simulink model "Integral_controller_disturbance"  (R2018b)
settings: Solver=VariableStepAuto  StartTime=0.0  StopTime=10  MaxStep=1e-3  RelTol=1e-3
InitFcn:
  | % NOTE: If using VoltPAQ-X1, make sure both Gain switches are set to 3.
  | K_AMP = 3;
  | % Maximum Output Voltage (V): YAW limited to 15 V. PITCH limited to 24 V.
  | VMAX_AMP_P = 24;
  | VMAX_AMP_Y = 15;
  | % Initial Angle of Pitch (rad)
  | theta_0 = -40.5*pi/180;
  | 
  | g = 9.81;
  | 
  | % Pitch and Yaw Motor Armature Resistance (Ohm)
  | R_m_p = 0.83;
  | R_m_y = 1.60;
  | 
  | % Pitch and Yaw Motor Current-Torque Constant (N.m/A)
  | K_t_p = 0.0182;
  | K_t_y = 0.0109;
  | 
  | % Pitch and Yaw Motor Voltage-Torque Constant (N.m/V)
  | K_yp = K_t_p / R_m_p;
  | K_py = K_t_y / R_m_y;
  | 
  | % Pitch and Yaw Viscous Damping Constant (N.m.s/rad)
  | B_p = 0.8;  % tuned while running simulation and experiment in parallel
  | B_y = 0.318; % identified as described in manual
  | 
  | % Mass of the Helicopter (kg)
  | m_heli = 1.3872;
  | 
  | % Mass of the Helicopter with Yoke (kg)
  | m_heli_case = 1.421;
  | 
  | % Distance from Pitch Pivot to Pitch/Front Motor and Yaw/Back Motor(m)
  | r_p = 7.75*0.0254;
  | r_y = (6+5/8)*0.0254;
  | 
  | % Pitch and Yaw Propeller Force-Thrust Constant found Experimentally (N/V)
  | K_f_p = 5*0.2074;
  | K_f_y = 3*0.1426;
  | 
  | % Pitch and Yaw Propeller Torque-Thrust Constant found Experimentally (N.m/V)
  | K_pp = K_f_p * r_p;
  | K_yy = K_f_y * r_y;
  | 
  | % Mass of Pitch/Front Motor and Yaw/Back Motor (kg)
  | m_motor_p = 0.292;
  | m_motor_y = 0.128;
  | 
  | % Mass of Pitch/Front and Yaw/Back Guard + Propeller(kg)
  | m_shield = 0.143 + 0.024;
  | 
  | % Total Mass of Pitch and Yaw Motor/Shield Assemblies (kg)
  | m_props = ( m_motor_p + m_motor_y + 2 * m_shield );
  | 
  | % Mass of Helicopter Body moving about Pitch Axis (kg)
  | m_body_p = m_heli - m_props;
  | 
  | % Mass of Helicopter Body moving about Yaw Axis (kg)
  | m_body_y = m_heli_case - m_props;
  | 
  | % Mass of Metal Shaft Moving about Yaw Axis (kg)
  | m_shaft = 0.151;
  | 
  | % Total Length of Helicopter Body (m)
  | L_body = 19*0.0254;
  | 
  | % Helicopter Center of Mass from Pivot along Pitch Axis (m)
  | l_cm = ( (m_motor_p + m_shield ) * r_p +  (m_motor_y + m_shield ) * r_y ) / ( m_props ) ;
  | 
  | % Length of Metal Shaft Moving about Yaw Axis through slip ring (m)
  | L_shaft = 11 * 0.0254;
  | 
  | % Pitch and Yaw Motor Rotor Moment of Inertia (kg.m^2)
  | J_m_p = 1.91e-6; %1.7070e-5;
  | J_m_y = 1.374e-4; %1.4471e-5;
  | 
  | % Moment of Inertia of Helicopter Body about its CM (kg.m^2)
  | J_body_p = m_body_p * L_body^2 / 12;
  | J_body_y = m_body_y * L_body^2 / 12;
  | 
  | % Moment of Inertia of Metal Shaft about Yaw Axis (kg.m^2)
  | J_shaft = m_shaft * L_shaft^2 / 3; %;0.0851;
  | 
  | % Moment of Inertia of Pitch Motor + Guard Assembly about Pivot (kg.m^2)
  | J_p = ( m_motor_p + m_shield ) * r_p^2;
  | 
  | % Moment of Inertia of Yaw Motor + Guard Assembly about Pivot (kg.m^2)
  | J_y = ( m_motor_y + m_shield ) * r_y^2;
  | 
  | % Equivalent Moment of Inertia about Pitch and Yaw Axis (kg.m^2)
  | J_eq_p = J_m_p + J_body_p + J_p + J_y;
  | J_eq_y = J_m_y + J_body_y + J_p + J_y + J_shaft;
  | 
  | 
  | %BESSEL wn=4
  | Kbes=[     68.5119  -25.1203    5.3421   -3.6881
  |    63.1652  188.4894    0.7783   19.4789];
  | 
  | xd=-20;
libraries: simulink x1
settings Model: Creator=rezan  LastModifiedBy=rezan
settings DataIOCC: ReturnWorkspaceOutputs=on
settings DebuggingCC: UnconnectedInputMsg=none  UnconnectedOutputMsg=none  UnconnectedLineMsg=none  SFMachineParentedDataDiag=error

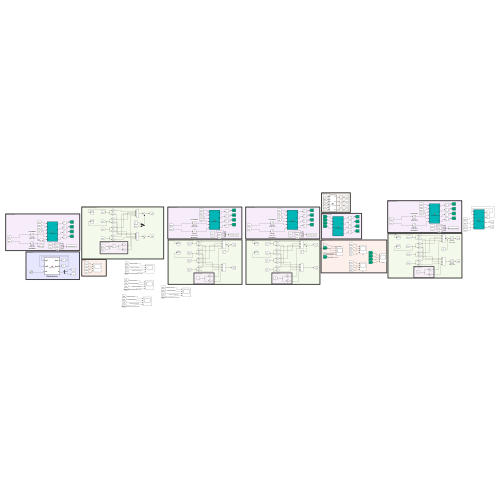
[thumbnail: Simulink's stored preview of the top-level diagram]
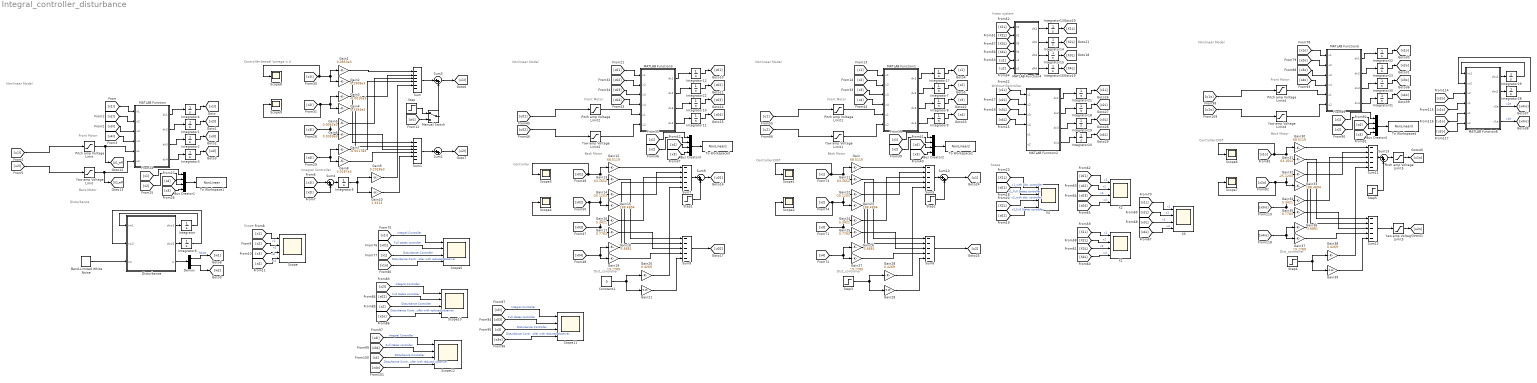
== system Integral_controller_disturbance ==
  note: Scope
  note: Disturbance
  note: Integral Controller
  note: Controller-bessel \omega = 4
  note: Front Motor
  note: Back Motor
  note: Nonlinear Model
  note: Controller-DIST
  note: Back Motor
  note: Dist_controller
  note: Scope
  note: Nonlinear Model
  note: Front Motor
  note: linear system
  note: Without Controller
  note: Dist_controller
  note: Controller
  note: Back Motor
  note: Nonlinear Model
  note: Front Motor
  note: Controller-DIST
  note: Dist_controller
  note: Front Motor
  note: Back Motor
  note: Nonlinear Model
  Band-Limited White Noise : simulink/Sources/Band-Limited White Noise  Cov=5  Ts=0.1  seed=[23341]
  Bus Creator{1..4} (4 alike) : BusCreator  Inputs=4
  Constant1 : Constant  Value=0
  Demux : Demux  Outputs=2
  Disturbance : MATLAB Function  TreatAsAtomicUnit=on
  Gain : Gain  Gain=68.5119
  Gain1 : Gain  Gain=0.0853e3
  Gain10 : Gain  Gain=1.3313
  Gain11 : Gain  Gain=63.1652
  Gain12 : Gain  Gain=68.5119
  Gain13 : Gain  Gain=63.1652
  Gain14 : Gain  Gain=-25.1203
  Gain15 : Gain  Gain=188.4894
  Gain16 : Gain  Gain=5.3421
  Gain17 : Gain  Gain=0.7783
  Gain18 : Gain  Gain=-3.6881
  Gain19 : Gain  Gain=19.4789
  Gain2 : Gain  Gain=0.1908e3
  Gain20 : Gain  Gain=0.4269
  Gain21 : Gain  Gain=-0.13
  Gain22 : Gain  Gain=-25.1203
  Gain23 : Gain  Gain=188.4894
  Gain24 : Gain  Gain=5.3421
  Gain25 : Gain  Gain=0.7783
  Gain26 : Gain  Gain=-3.6881
  Gain27 : Gain  Gain=19.4789
  Gain28 : Gain  Gain=0.4269
  Gain29 : Gain  Gain=-0.13
  Gain3 : Gain  Gain=-0.0010e3
  Gain30 : Gain  Gain=68.5119
  Gain31 : Gain  Gain=63.1652
  Gain32 : Gain  Gain=-25.1203
  Gain33 : Gain  Gain=188.4894
  Gain34 : Gain  Gain=5.3421
  Gain35 : Gain  Gain=0.7783
  Gain36 : Gain  Gain=-3.6881
  Gain37 : Gain  Gain=19.4789
  Gain38 : Gain  Gain=0.4269
  Gain39 : Gain  Gain=-0.13
  Gain4 : Gain  Gain=0.3394e3
  Gain5 : Gain  Gain=0.0061e3
  Gain6 : Gain  Gain=0.0059e3
  Gain7 : Gain  Gain=-0.0017e3
  Gain8 : Gain  Gain=0.0287e3
  Gain9 : Gain  Gain=0.2028e3
  Integrator{,1,3,6..7,9,11,14,16,18,20,22..23,28..29,31} (16 alike) : Integrator
  Integrator{2,8,10,15,19,30} (6 alike) : Integrator  InitialCondition=10
  Integrator{4..5,12..13,17,21,32} (7 alike) : Integrator  UpperSaturationLimit=40.5*pi/180  LowerSaturationLimit=-40.5*pi/180
  MATLAB Function : MATLAB Function  TreatAsAtomicUnit=on
  MATLAB Function1 : MATLAB Function  TreatAsAtomicUnit=on
  MATLAB Function2 : MATLAB Function  TreatAsAtomicUnit=on
  MATLAB Function3 : MATLAB Function  TreatAsAtomicUnit=on
  MATLAB Function4 : MATLAB Function  TreatAsAtomicUnit=on
  MATLAB Function5 : MATLAB Function  TreatAsAtomicUnit=on
  MATLAB Function8 : MATLAB Function  TreatAsAtomicUnit=on
  Manual Switch : ManualSwitch
  Pitch amp Voltage Limit{,1..2,4..5} (5 alike) : Saturate  UpperLimit=VMAX_AMP_P  LowerLimit=- VMAX_AMP_P
  Scope{,5,10..12} (5 alike) : Scope  NumInputPorts=4
  Scope{1..4,6..9} (8 alike) : Scope
  Step{,1..5} (6 alike) : Step  SampleTime=0
  Sum : Sum  Inputs=------
  Sum1 : Sum  Inputs=------
  Sum{2..4,9..10,13} (6 alike) : Sum  Inputs=|++
  Sum{5..8,11..12} (6 alike) : Sum  Inputs=-----
  To Workspace1 : ToWorkspace  VariableName=NonLinear  SampleTime=-1
  To Workspace2 : ToWorkspace  VariableName=NonLinear2  SampleTime=-1
  To Workspace3 : ToWorkspace  VariableName=NonLinear1  SampleTime=-1
  To Workspace4 : ToWorkspace  VariableName=NonLinear3  SampleTime=-1
  X{1..4} (4 alike) : Scope  NumInputPorts=4
  Yaw amp Voltage Limit{,1..2,4..5} (5 alike) : Saturate  UpperLimit=VMAX_AMP_Y  LowerLimit=- VMAX_AMP_Y
  wires:
  Sum1/1 -> Sum2/1
  Gain4/1 -> Sum1/2
  [x2I] -> Scope9/1, Gain3/1, Gain4/1
  Integrator5/1 -> Gain10/1, Gain9/1
  Gain6/1 -> Sum1/3
  Sum3/1 -> [u1I]
  Gain7/1 -> Sum/4
  [x4I] -> Gain8/1, Gain7/1
  Gain2/1 -> Sum1/1
  Gain9/1 -> Sum/5
  Gain5/1 -> Sum/3
  [x3I] -> Gain5/1, Gain6/1
  Sum2/1 -> [u2I]
  Sum/1 -> Sum3/1
  Gain1/1 -> Sum/1
  Gain8/1 -> Sum1/4
  [x1I] -> Scope8/1, Gain2/1, Gain1/1
  Gain10/1 -> Sum1/5
  Gain3/1 -> Sum/2
  MATLAB Function/3(dx3) -> Integrator2/1
  Integrator4/1 -> [x1I]
  [x2] -> Bus Creator1/2
  Pitch amp Voltage Limit/1 -> [U1_eff], MATLAB Function/5(u1)
  Bus Creator1/1 -> To Workspace1/1
  [x4] -> Bus Creator1/3
  [x3I] -> MATLAB Function/3(x3)
  Integrator2/1 -> [x3I]
  MATLAB Function/1(dx1) -> Integrator4/1
  MATLAB Function/4(dx4) -> Integrator3/1
  MATLAB Function/2(dx2) -> Integrator1/1
  [x2I] -> MATLAB Function/2(x2)
  [u1I] -> Pitch amp Voltage Limit/1
  Integrator3/1 -> [x4I]
  [u2I] -> Yaw amp Voltage Limit/1
  [x4I] -> MATLAB Function/4(x4)
  [x3] -> Bus Creator1/4
  [x1] -> Bus Creator1/1
  Integrator1/1 -> [x2I]
  Yaw amp Voltage Limit/1 -> [U2_eff], MATLAB Function/6(u2)
  [x1I] -> MATLAB Function/1(x1)
  [x1I] -> Sum4/1
  [x2I] -> Sum4/2
  Sum4/1 -> Integrator5/1
  [x1] -> Scope/1  "x1"
  [x2] -> Scope/2  "x2"
  [x3] -> Scope/3  "x3"
  [x4] -> Scope/4  "x4"
  Disturbance/1(dxw1) -> Integrator/1
  Band-Limited White Noise/1 -> Disturbance/3(uw)
  Integrator/1 -> Disturbance/1(xw1)
  Disturbance/2(dxw2) -> Integrator6/1
  Integrator6/1 -> Disturbance/2(xw2)
  Demux/1 -> [w1]  "Noise"
  Disturbance/3(w) -> Demux/1
  Demux/2 -> [w2]
  Step/1 -> Manual Switch/1
  [w1] -> Manual Switch/2
  Manual Switch/1 -> Sum3/2
  [X2L] -> MATLAB Function4/2(X2)
  [x1] -> Bus Creator3/1
  Integrator15/1 -> [X3L]
  Sum10/1 -> [u1]
  Integrator14/1 -> [X2L]
  [u1] -> MATLAB Function4/5(u1)
  [x4] -> MATLAB Function1/4(x4)
  [x04] -> MATLAB Function3/4(x4)
  [X1L] -> MATLAB Function4/1(X1)
  [X2L] -> X1/2  "x2"
  [x3] -> Bus Creator3/4
  Gain17/1 -> Sum8/3
  Yaw amp Voltage Limit1/1 -> MATLAB Function1/6(u2)
  Integrator16/1 -> [X4L]
  Integrator13/1 -> [X1L]
  Integrator10/1 -> [x03]
  Integrator12/1 -> [x01]
  [x02] -> X4/4  "x2_Full States controller"
  MATLAB Function2/1(dx1) -> Integrator21/1
  Integrator21/1 -> [x1L]
  Gain22/1 -> Sum5/2
  [x01] -> Gain12/1, Gain13/1, Scope3/1
  [x2] -> Scope2/1, Gain22/1, Gain23/1
  Constant1/1 -> Gain20/1, Gain21/1
  MATLAB Function4/2(dX2) -> Integrator14/1
  Bus Creator3/1 -> To Workspace3/1
  [X4L] -> MATLAB Function4/4(X4)
  Gain12/1 -> Sum7/1
  [x1L] -> MATLAB Function2/1(x1)
  [X3L] -> MATLAB Function4/3(X3)
  MATLAB Function4/1(dX1) -> Integrator13/1
  Integrator22/1 -> [x02]
  [u01] -> Pitch amp Voltage Limit2/1
  [x4] -> Bus Creator3/3
  [x01] -> MATLAB Function3/1(x1)
  Yaw amp Voltage Limit2/1 -> MATLAB Function3/6(u2)
  [u02] -> Yaw amp Voltage Limit2/1
  [x2] -> MATLAB Function1/2(x2)
  Integrator11/1 -> [x04]
  MATLAB Function3/3(dx3) -> Integrator10/1
  [x3] -> MATLAB Function1/3(x3)
  Integrator20/1 -> [x4L]
  MATLAB Function1/4(dx4) -> Integrator9/1
  [x04] -> Gain18/1, Gain19/1
  MATLAB Function3/2(dx2) -> Integrator22/1
  [x03] -> MATLAB Function3/3(x3)
  Gain13/1 -> Sum8/1
  Gain18/1 -> Sum7/4
  Gain15/1 -> Sum8/2
  MATLAB Function3/1(dx1) -> Integrator12/1
  Gain16/1 -> Sum7/3
  [x02] -> Gain15/1, Gain14/1, Scope4/1
  Gain27/1 -> Sum6/4
  Sum8/1 -> [u02]
  MATLAB Function2/4(dx4) -> Integrator20/1
  MATLAB Function1/3(dx3) -> Integrator8/1
  Bus Creator2/1 -> To Workspace2/1
  MATLAB Function2/3(dx3) -> Integrator19/1
  Integrator19/1 -> [x3L]
  [x3L] -> MATLAB Function2/3(x3)
  Gain11/1 -> Sum6/1
  [x4L] -> MATLAB Function2/4(x4)
  [x4] -> Gain27/1, Gain26/1
  Gain28/1 -> Sum5/5
  Gain25/1 -> Sum6/3
  MATLAB Function4/4(dX4) -> Integrator16/1
  [u1] -> Pitch amp Voltage Limit1/1
  Integrator18/1 -> [x2L]
  [x1] -> Scope1/1, Gain11/1, Gain/1
  Integrator9/1 -> [x4]
  [x2] -> Bus Creator3/2
  Gain/1 -> Sum5/1
  [x2] -> Bus Creator2/2
  MATLAB Function2/2(dx2) -> Integrator18/1
  [X2L] -> X4/3  "x2_with dist. controller"
  [x1] -> Bus Creator2/1
  [x3] -> Gain24/1, Gain25/1
  MATLAB Function1/1(dx1) -> Integrator17/1
  [x1] -> MATLAB Function1/1(x1)
  [X3L] -> X1/3  "x3"
  [X1L] -> X4/1  "x1_with dist. controller"
  [u2] -> Yaw amp Voltage Limit1/1
  Integrator8/1 -> [x3]
  [x02] -> X2/2  "x2"
  [x03] -> X2/3  "x3"
  Pitch amp Voltage Limit1/1 -> MATLAB Function1/5(u1)
  Gain19/1 -> Sum8/4
  [x01] -> X2/1  "x1"
  [X1L] -> X1/1  "x1"
  MATLAB Function4/3(dX3) -> Integrator15/1
  Gain29/1 -> Sum6/5
  Integrator7/1 -> [x2]
  [x01] -> X4/2  "x1_Full States controller"
  MATLAB Function3/4(dx4) -> Integrator11/1
  Gain26/1 -> Sum5/4
  [x02] -> MATLAB Function3/2(x2)
  Gain14/1 -> Sum7/2
  Gain23/1 -> Sum6/2
  [x4L] -> X3/4  "x4"
  [X4L] -> X1/4  "x4"
  Step3/1 -> Gain29/1, Gain28/1
  Gain20/1 -> Sum7/5
  Integrator17/1 -> [x1]
  Sum6/1 -> [u2]
  Gain24/1 -> Sum5/3
  [x1L] -> X3/1  "x1"
  MATLAB Function1/2(dx2) -> Integrator7/1
  [x03] -> Gain17/1, Gain16/1
  [x04] -> X2/4  "x4"
  Gain21/1 -> Sum8/5
  [x4] -> Bus Creator2/3
  [x2L] -> X3/2  "x2"
  [x3L] -> X3/3  "x3"
  [x3] -> Bus Creator2/4
  Pitch amp Voltage Limit2/1 -> MATLAB Function3/5(u1)
  [x2L] -> MATLAB Function2/2(x2)
  [u2] -> MATLAB Function4/6(u2)
  Step1/1 -> Sum9/2
  Sum9/1 -> [u01]
  Sum7/1 -> Sum9/1
  Sum5/1 -> Sum10/1
  Step2/1 -> Sum10/2
  [x1I] -> Scope5/1  "Integral Controller"
  [x01] -> Scope5/2  "Full states controller"
  [x1] -> Scope5/3  "Disturbance Controller"
  Step4/1 -> Gain39/1, Gain38/1
  Gain38/1 -> Sum11/5
  [x4o] -> MATLAB Function5/4(x4)
  [x2o] -> Scope7/1, Gain32/1, Gain33/1
  Integrator30/1 -> [x3o]
  [x3o] -> MATLAB Function5/3(x3)
  [x1o] -> Scope6/1, Gain31/1, Gain30/1
  [u1o] -> Pitch amp Voltage Limit4/1
  MATLAB Function5/2(dx2) -> Integrator23/1
  Integrator31/1 -> [x4o]
  Integrator32/1 -> [x1o]
  Sum12/1 -> Yaw amp Voltage Limit5/1
  Gain35/1 -> Sum12/3
  Gain33/1 -> Sum12/2
  Gain34/1 -> Sum11/3
  Gain30/1 -> Sum11/1
  [x3ro] -> Gain34/1, Gain35/1
  Gain39/1 -> Sum12/5
  [x2o] -> MATLAB Function8/3(x2)
  [u2o] -> MATLAB Function8/6(u2)
  Gain36/1 -> Sum11/4
  Integrator28/1 -> MATLAB Function8/2(xc2)
  [x2] -> Bus Creator4/2
  MATLAB Function8/1(dxc1) -> Integrator29/1
  Integrator29/1 -> MATLAB Function8/1(xc1)
  [x4ro] -> Gain37/1, Gain36/1
  MATLAB Function8/2(dxc2) -> Integrator28/1
  MATLAB Function5/4(dx4) -> Integrator31/1
  MATLAB Function5/1(dx1) -> Integrator32/1
  Yaw amp Voltage Limit4/1 -> MATLAB Function5/6(u2)
  [x3] -> Bus Creator4/4
  MATLAB Function5/3(dx3) -> Integrator30/1
  Gain32/1 -> Sum11/2
  Pitch amp Voltage Limit5/1 -> [u1o]
  MATLAB Function8/4(x1e) -> [x3ro]  "x1e"
  Yaw amp Voltage Limit5/1 -> [u2o]
  [x1] -> Bus Creator4/1
  [u1o] -> MATLAB Function8/5(u1)
  Integrator23/1 -> [x2o]
  [x1o] -> MATLAB Function8/4(x1)
  [x2o] -> MATLAB Function5/2(x2)
  [u2o] -> Yaw amp Voltage Limit4/1
  [x1o] -> MATLAB Function5/1(x1)
  Gain37/1 -> Sum12/4
  MATLAB Function8/3(x2e) -> [x4ro]  "x2e"
  [x4] -> Bus Creator4/3
  Bus Creator4/1 -> To Workspace4/1
  Pitch amp Voltage Limit4/1 -> MATLAB Function5/5(u1)
  Gain31/1 -> Sum12/1
  Step5/1 -> Sum13/2
  Sum11/1 -> Sum13/1
  Sum13/1 -> Pitch amp Voltage Limit5/1
  [x1o] -> Scope5/4  "Disturbance Controller with reduced observer"
  [x2o] -> Scope10/4  "Disturbance Controller with reduced observer"
  [x2] -> Scope10/3  "Disturbance Controller"
  [x02] -> Scope10/2  "Full states controller"
  [x2I] -> Scope10/1  "Integral Controller"
  [x3I] -> Scope11/1  "Integral Controller"
  [x03] -> Scope11/2  "Full states controller"
  [x3] -> Scope11/3  "Disturbance Controller"
  [x3o] -> Scope11/4  "Disturbance Controller with reduced observer"
  [x4o] -> Scope12/4  "Disturbance Controller with reduced observer"
  [x4] -> Scope12/3  "Disturbance Controller"
  [x04] -> Scope12/2  "Full states controller"
  [x4I] -> Scope12/1  "Integral Controller"

== matlab function Integral_controller_disturbance/MATLAB Function1 ==
  data: x1 input; x2 input; x3 input; x4 input; u1 input; dx1 output; u2 input; dx2 output; dx3 output; dx4 output
function [dx1,dx2,dx3,dx4]= NonlinearFunc(x1,x2,x3,x4,u1,u2)
%% Initial Conditions
% Gravitational Constant (m/s^2)
g = 9.81;

% Pitch and Yaw Motor Armature Resistance (Ohm)
R_m_p = 0.83;
R_m_y = 1.60;

% Pitch and Yaw Motor Current-Torque Constant (N.m/A)
K_t_p = 0.0182;
K_t_y = 0.0109;

% Pitch and Yaw Motor Voltage-Torque Constant (N.m/V)
K_yp = K_t_p / R_m_p;
K_py = K_t_y / R_m_y;

% Pitch and Yaw Viscous Damping Constant (N.m.s/rad)
B_p = 0.8;  % tuned while running simulation and experiment in parallel
B_y = 0.318; % identified as described in manual 

% Mass of the Helicopter (kg)
m_heli = 1.3872;

% Mass of the Helicopter with Yoke (kg)
m_heli_case = 1.421;

% Distance from Pitch Pivot to Pitch/Front Motor and Yaw/Back Motor(m)
r_p = 7.75*0.0254;
r_y = (6+5/8)*0.0254;

% Pitch and Yaw Propeller Force-Thrust Constant found Experimentally (N/V)
K_f_p = 5*0.2074;
K_f_y = 3*0.1426;

% Pitch and Yaw Propeller Torque-Thrust Constant found Experimentally (N.m/V)
K_pp = K_f_p * r_p;
K_yy = K_f_y * r_y;

% Mass of Pitch/Front Motor and Yaw/Back Motor (kg)
m_motor_p = 0.292;
m_motor_y = 0.128;

% Mass of Pitch/Front and Yaw/Back Guard + Propeller(kg)
m_shield = 0.143 + 0.024;

% Total Mass of Pitch and Yaw Motor/Shield Assemblies (kg)
m_props = ( m_motor_p + m_motor_y + 2 * m_shield );

% Mass of Helicopter Body moving about Pitch Axis (kg)
m_body_p = m_heli - m_props; 

% Mass of Helicopter Body moving about Yaw Axis (kg)
m_body_y = m_heli_case - m_props; 

% Mass of Metal Shaft Moving about Yaw Axis (kg)
m_shaft = 0.151;

% Total Length of Helicopter Body (m)
L_body = 19*0.0254;

% Helicopter Center of Mass from Pivot along Pitch Axis (m)
l_cm = ( (m_motor_p + m_shield ) * r_p +  (m_motor_y + m_shield ) * r_y ) / ( m_props ) ;

% Length of Metal Shaft Moving about Yaw Axis through slip ring (m)
L_shaft = 11 * 0.0254;

% Pitch and Yaw Motor Rotor Moment of Inertia (kg.m^2)
J_m_p = 1.91e-6; %1.7070e-5;
J_m_y = 1.374e-4; %1.4471e-5;

% Moment of Inertia of Helicopter Body about its CM (kg.m^2)
J_body_p = m_body_p * L_body^2 / 12;
J_body_y = m_body_y * L_body^2 / 12;

% Moment of Inertia of Metal Shaft about Yaw Axis (kg.m^2)
J_shaft = m_shaft * L_shaft^2 / 3; %;0.0851;

% Moment of Inertia of Pitch Motor + Guard Assembly about Pivot (kg.m^2)
J_p = ( m_motor_p + m_shield ) * r_p^2;

% Moment of Inertia of Yaw Motor + Guard Assembly about Pivot (kg.m^2)
J_y = ( m_motor_y + m_shield ) * r_y^2;

% Equivalent Moment of Inertia about Pitch and Yaw Axis (kg.m^2)
J_eq_p = J_m_p + J_body_p + J_p + J_y;
J_eq_y = J_m_y + J_body_y + J_p + J_y + J_shaft;
%%
%%
xd=0
 dx1=x3;
dx2=x4;
dx3=(1/(J_eq_p +m_heli*l_cm^2))*((K_pp*u1+K_py*u2)-(B_p*x3+m_heli*l_cm^2*x4^2*sin(x1)*cos(x1)+m_heli*g*l_cm*cos(x1)));
dx3=dx3+xd;
dx4=1/(J_eq_y + m_heli *l_cm^2* (cos(x1))^2 )*((K_yp*u1 )+(K_yy*u2 ))+(-B_y*x4+2*m_heli*l_cm^2*x4*x3*sin(x1)*cos(x1))/(J_eq_p+ m_heli * l_cm^2 * (cos(x1))^2);

== matlab function Integral_controller_disturbance/MATLAB Function2 ==
  data: x1 input; x2 input; x3 input; x4 input; u1 input; dx1 output; u2 input; dx2 output; dx3 output; dx4 output
function [dx1,dx2,dx3,dx4]= NonlinearFunc(x1,x2,x3,x4,u1,u2)
%% Initial Conditions
% Gravitational Constant (m/s^2)
g = 9.81;

% Pitch and Yaw Motor Armature Resistance (Ohm)
R_m_p = 0.83;
R_m_y = 1.60;

% Pitch and Yaw Motor Current-Torque Constant (N.m/A)
K_t_p = 0.0182;
K_t_y = 0.0109;

% Pitch and Yaw Motor Voltage-Torque Constant (N.m/V)
K_yp = K_t_p / R_m_p;
K_py = K_t_y / R_m_y;

% Pitch and Yaw Viscous Damping Constant (N.m.s/rad)
B_p = 0.8;  % tuned while running simulation and experiment in parallel
B_y = 0.318; % identified as described in manual 

% Mass of the Helicopter (kg)
m_heli = 1.3872;

% Mass of the Helicopter with Yoke (kg)
m_heli_case = 1.421;

% Distance from Pitch Pivot to Pitch/Front Motor and Yaw/Back Motor(m)
r_p = 7.75*0.0254;
r_y = (6+5/8)*0.0254;

% Pitch and Yaw Propeller Force-Thrust Constant found Experimentally (N/V)
K_f_p = 5*0.2074;
K_f_y = 3*0.1426;

% Pitch and Yaw Propeller Torque-Thrust Constant found Experimentally (N.m/V)
K_pp = K_f_p * r_p;
K_yy = K_f_y * r_y;

% Mass of Pitch/Front Motor and Yaw/Back Motor (kg)
m_motor_p = 0.292;
m_motor_y = 0.128;

% Mass of Pitch/Front and Yaw/Back Guard + Propeller(kg)
m_shield = 0.143 + 0.024;

% Total Mass of Pitch and Yaw Motor/Shield Assemblies (kg)
m_props = ( m_motor_p + m_motor_y + 2 * m_shield );

% Mass of Helicopter Body moving about Pitch Axis (kg)
m_body_p = m_heli - m_props; 

% Mass of Helicopter Body moving about Yaw Axis (kg)
m_body_y = m_heli_case - m_props; 

% Mass of Metal Shaft Moving about Yaw Axis (kg)
m_shaft = 0.151;

% Total Length of Helicopter Body (m)
L_body = 19*0.0254;

% Helicopter Center of Mass from Pivot along Pitch Axis (m)
l_cm = ( (m_motor_p + m_shield ) * r_p +  (m_motor_y + m_shield ) * r_y ) / ( m_props ) ;

% Length of Metal Shaft Moving about Yaw Axis through slip ring (m)
L_shaft = 11 * 0.0254;

% Pitch and Yaw Motor Rotor Moment of Inertia (kg.m^2)
J_m_p = 1.91e-6; %1.7070e-5;
J_m_y = 1.374e-4; %1.4471e-5;

% Moment of Inertia of Helicopter Body about its CM (kg.m^2)
J_body_p = m_body_p * L_body^2 / 12;
J_body_y = m_body_y * L_body^2 / 12;

% Moment of Inertia of Metal Shaft about Yaw Axis (kg.m^2)
J_shaft = m_shaft * L_shaft^2 / 3; %;0.0851;

% Moment of Inertia of Pitch Motor + Guard Assembly about Pivot (kg.m^2)
J_p = ( m_motor_p + m_shield ) * r_p^2;

% Moment of Inertia of Yaw Motor + Guard Assembly about Pivot (kg.m^2)
J_y = ( m_motor_y + m_shield ) * r_y^2;

% Equivalent Moment of Inertia about Pitch and Yaw Axis (kg.m^2)
J_eq_p = J_m_p + J_body_p + J_p + J_y;
J_eq_y = J_m_y + J_body_y + J_p + J_y + J_shaft;
%%
%%
xd=0
 dx1=x3;
dx2=x4;
dx3=(1/(J_eq_p +m_heli*l_cm^2))*((K_pp*u1+K_py*u2)-(B_p*x3+m_heli*l_cm^2*x4^2*sin(x1)*cos(x1)+m_heli*g*l_cm*cos(x1)));
dx3=dx3+xd;
dx4=1/(J_eq_y + m_heli *l_cm^2* (cos(x1))^2 )*((K_yp*u1 )+(K_yy*u2 ))+(-B_y*x4+2*m_heli*l_cm^2*x4*x3*sin(x1)*cos(x1))/(J_eq_p+ m_heli * l_cm^2 * (cos(x1))^2);

== matlab function Integral_controller_disturbance/MATLAB Function3 ==
  data: x1 input; x2 input; x3 input; x4 input; u1 input; dx1 output; u2 input; dx2 output; dx3 output; dx4 output
function [dx1,dx2,dx3,dx4]= NonlinearFunc(x1,x2,x3,x4,u1,u2)
%% Initial Conditions
% Gravitational Constant (m/s^2)
g = 9.81;

% Pitch and Yaw Motor Armature Resistance (Ohm)
R_m_p = 0.83;
R_m_y = 1.60;

% Pitch and Yaw Motor Current-Torque Constant (N.m/A)
K_t_p = 0.0182;
K_t_y = 0.0109;

% Pitch and Yaw Motor Voltage-Torque Constant (N.m/V)
K_yp = K_t_p / R_m_p;
K_py = K_t_y / R_m_y;

% Pitch and Yaw Viscous Damping Constant (N.m.s/rad)
B_p = 0.8;  % tuned while running simulation and experiment in parallel
B_y = 0.318; % identified as described in manual 

% Mass of the Helicopter (kg)
m_heli = 1.3872;

% Mass of the Helicopter with Yoke (kg)
m_heli_case = 1.421;

% Distance from Pitch Pivot to Pitch/Front Motor and Yaw/Back Motor(m)
r_p = 7.75*0.0254;
r_y = (6+5/8)*0.0254;

% Pitch and Yaw Propeller Force-Thrust Constant found Experimentally (N/V)
K_f_p = 5*0.2074;
K_f_y = 3*0.1426;

% Pitch and Yaw Propeller Torque-Thrust Constant found Experimentally (N.m/V)
K_pp = K_f_p * r_p;
K_yy = K_f_y * r_y;

% Mass of Pitch/Front Motor and Yaw/Back Motor (kg)
m_motor_p = 0.292;
m_motor_y = 0.128;

% Mass of Pitch/Front and Yaw/Back Guard + Propeller(kg)
m_shield = 0.143 + 0.024;

% Total Mass of Pitch and Yaw Motor/Shield Assemblies (kg)
m_props = ( m_motor_p + m_motor_y + 2 * m_shield );

% Mass of Helicopter Body moving about Pitch Axis (kg)
m_body_p = m_heli - m_props; 

% Mass of Helicopter Body moving about Yaw Axis (kg)
m_body_y = m_heli_case - m_props; 

% Mass of Metal Shaft Moving about Yaw Axis (kg)
m_shaft = 0.151;

% Total Length of Helicopter Body (m)
L_body = 19*0.0254;

% Helicopter Center of Mass from Pivot along Pitch Axis (m)
l_cm = ( (m_motor_p + m_shield ) * r_p +  (m_motor_y + m_shield ) * r_y ) / ( m_props ) ;

% Length of Metal Shaft Moving about Yaw Axis through slip ring (m)
L_shaft = 11 * 0.0254;

% Pitch and Yaw Motor Rotor Moment of Inertia (kg.m^2)
J_m_p = 1.91e-6; %1.7070e-5;
J_m_y = 1.374e-4; %1.4471e-5;

% Moment of Inertia of Helicopter Body about its CM (kg.m^2)
J_body_p = m_body_p * L_body^2 / 12;
J_body_y = m_body_y * L_body^2 / 12;

% Moment of Inertia of Metal Shaft about Yaw Axis (kg.m^2)
J_shaft = m_shaft * L_shaft^2 / 3; %;0.0851;

% Moment of Inertia of Pitch Motor + Guard Assembly about Pivot (kg.m^2)
J_p = ( m_motor_p + m_shield ) * r_p^2;

% Moment of Inertia of Yaw Motor + Guard Assembly about Pivot (kg.m^2)
J_y = ( m_motor_y + m_shield ) * r_y^2;

% Equivalent Moment of Inertia about Pitch and Yaw Axis (kg.m^2)
J_eq_p = J_m_p + J_body_p + J_p + J_y;
J_eq_y = J_m_y + J_body_y + J_p + J_y + J_shaft;
%%
%%
xd=-0
 dx1=x3;
dx2=x4;
dx3=(1/(J_eq_p +m_heli*l_cm^2))*((K_pp*u1+K_py*u2)-(B_p*x3+m_heli*l_cm^2*x4^2*sin(x1)*cos(x1)+m_heli*g*l_cm*cos(x1)));
dx3=dx3+xd;
dx4=1/(J_eq_y + m_heli *l_cm^2* (cos(x1))^2 )*((K_yp*u1 )+(K_yy*u2 ))+(-B_y*x4+2*m_heli*l_cm^2*x4*x3*sin(x1)*cos(x1))/(J_eq_p+ m_heli * l_cm^2 * (cos(x1))^2);

== matlab function Integral_controller_disturbance/MATLAB Function4 ==
  data: X1 input; dX1 output; X2 input; X3 input; X4 input; u1 input; dX2 output; dX3 output; dX4 output; u2 input
function [dX1,dX2,dX3,dX4] = Linear(X1,X2,X3,X4,u1,u2)
%#codegen

A=[      0         0    1.0000         0
         0         0         0    1.0000
         0         0   -9.2751         0
         0         0         0   -3.4955];
     
B=[      0         0
         0         0
    2.3667    0.0790
    0.2410    0.7913];

X = [X1;X2;X3;X4];
U=[u1,u2].';
dX = A*X+B*U;
xd=-30;

dX1 = dX(1);
dX2 = dX(2);
dX3 = dX(3)+0;
dX4 = dX(4);

== matlab function Integral_controller_disturbance/MATLAB Function5 ==
  data: x1 input; x2 input; x3 input; x4 input; u1 input; dx1 output; u2 input; dx2 output; dx3 output; dx4 output
function [dx1,dx2,dx3,dx4]= NonlinearFunc(x1,x2,x3,x4,u1,u2)
%% Initial Conditions
% Gravitational Constant (m/s^2)
g = 9.81;

% Pitch and Yaw Motor Armature Resistance (Ohm)
R_m_p = 0.83;
R_m_y = 1.60;

% Pitch and Yaw Motor Current-Torque Constant (N.m/A)
K_t_p = 0.0182;
K_t_y = 0.0109;

% Pitch and Yaw Motor Voltage-Torque Constant (N.m/V)
K_yp = K_t_p / R_m_p;
K_py = K_t_y / R_m_y;

% Pitch and Yaw Viscous Damping Constant (N.m.s/rad)
B_p = 0.8;  % tuned while running simulation and experiment in parallel
B_y = 0.318; % identified as described in manual 

% Mass of the Helicopter (kg)
m_heli = 1.3872;

% Mass of the Helicopter with Yoke (kg)
m_heli_case = 1.421;

% Distance from Pitch Pivot to Pitch/Front Motor and Yaw/Back Motor(m)
r_p = 7.75*0.0254;
r_y = (6+5/8)*0.0254;

% Pitch and Yaw Propeller Force-Thrust Constant found Experimentally (N/V)
K_f_p = 5*0.2074;
K_f_y = 3*0.1426;

% Pitch and Yaw Propeller Torque-Thrust Constant found Experimentally (N.m/V)
K_pp = K_f_p * r_p;
K_yy = K_f_y * r_y;

% Mass of Pitch/Front Motor and Yaw/Back Motor (kg)
m_motor_p = 0.292;
m_motor_y = 0.128;

% Mass of Pitch/Front and Yaw/Back Guard + Propeller(kg)
m_shield = 0.143 + 0.024;

% Total Mass of Pitch and Yaw Motor/Shield Assemblies (kg)
m_props = ( m_motor_p + m_motor_y + 2 * m_shield );

% Mass of Helicopter Body moving about Pitch Axis (kg)
m_body_p = m_heli - m_props; 

% Mass of Helicopter Body moving about Yaw Axis (kg)
m_body_y = m_heli_case - m_props; 

% Mass of Metal Shaft Moving about Yaw Axis (kg)
m_shaft = 0.151;

% Total Length of Helicopter Body (m)
L_body = 19*0.0254;

% Helicopter Center of Mass from Pivot along Pitch Axis (m)
l_cm = ( (m_motor_p + m_shield ) * r_p +  (m_motor_y + m_shield ) * r_y ) / ( m_props ) ;

% Length of Metal Shaft Moving about Yaw Axis through slip ring (m)
L_shaft = 11 * 0.0254;

% Pitch and Yaw Motor Rotor Moment of Inertia (kg.m^2)
J_m_p = 1.91e-6; %1.7070e-5;
J_m_y = 1.374e-4; %1.4471e-5;

% Moment of Inertia of Helicopter Body about its CM (kg.m^2)
J_body_p = m_body_p * L_body^2 / 12;
J_body_y = m_body_y * L_body^2 / 12;

% Moment of Inertia of Metal Shaft about Yaw Axis (kg.m^2)
J_shaft = m_shaft * L_shaft^2 / 3; %;0.0851;

% Moment of Inertia of Pitch Motor + Guard Assembly about Pivot (kg.m^2)
J_p = ( m_motor_p + m_shield ) * r_p^2;

% Moment of Inertia of Yaw Motor + Guard Assembly about Pivot (kg.m^2)
J_y = ( m_motor_y + m_shield ) * r_y^2;

% Equivalent Moment of Inertia about Pitch and Yaw Axis (kg.m^2)
J_eq_p = J_m_p + J_body_p + J_p + J_y;
J_eq_y = J_m_y + J_body_y + J_p + J_y + J_shaft;
%%
%%
xd=0
 dx1=x3;
dx2=x4;
dx3=(1/(J_eq_p +m_heli*l_cm^2))*((K_pp*u1+K_py*u2)-(B_p*x3+m_heli*l_cm^2*x4^2*sin(x1)*cos(x1)+m_heli*g*l_cm*cos(x1)));
dx3=dx3+xd;
dx4=1/(J_eq_y + m_heli *l_cm^2* (cos(x1))^2 )*((K_yp*u1 )+(K_yy*u2 ))+(-B_y*x4+2*m_heli*l_cm^2*x4*x3*sin(x1)*cos(x1))/(J_eq_p+ m_heli * l_cm^2 * (cos(x1))^2);

== matlab function Integral_controller_disturbance/MATLAB Function8 ==
  data: xc1 input; xc2 input; x2 input; x1 input; u1 input; dxc1 output; dxc2 output; x2e output; x1e output; u2 input
function [dxc1,dxc2,x2e,x1e] = Observer(xc1,xc2,x2,x1,u1,u2)

A=[      0         0    1.0000         0
         0         0         0    1.0000
         0         0   -9.2751         0
         0         0         0   -3.4955];
     
B=[      0         0
         0         0
    2.3667    0.0790
    0.2410    0.7913];
C=[  1     0     0     0
     0     1     0     0];

 D=[  0     0
     0     0];

 
C = eye(2,4);
Aee = A(3:4,3:4);
Aes = A(3:4,1:2);
Ase = A(1:2,3:4);
Ass = A(1:2,1:2);

Be = B(3:4,1);
Bs = B(1:2,1);

Cs = C(1:2,1:2);
L = [   -4.2751         0
         0    2.5045];
xc = [xc1;xc2];
y = [x1;x2];
xs = [x1;x2];
u=[u1,u2];
dxc = (Aee-L*Cs*Ase)*(xc+L*y)+(Aes*inv(Cs)-L*Cs*Ass*inv(Cs))*y+(Be-L*Cs*Bs)*u;
dxc1 = dxc(1);
dxc2 = dxc(2);
Xe = xc+L*y;
x1e = Xe(1);
x2e = Xe(2);

== matlab function Integral_controller_disturbance/MATLAB Function ==
  data: x1 input; x2 input; x3 input; x4 input; u1 input; dx1 output; u2 input; dx2 output; dx3 output; dx4 output
function [dx1,dx2,dx3,dx4]= NonlinearFunc(x1,x2,x3,x4,u1,u2)
%% Initial Conditions
% Gravitational Constant (m/s^2)
g = 9.81;

% Pitch and Yaw Motor Armature Resistance (Ohm)
R_m_p = 0.83;
R_m_y = 1.60;

% Pitch and Yaw Motor Current-Torque Constant (N.m/A)
K_t_p = 0.0182;
K_t_y = 0.0109;

% Pitch and Yaw Motor Voltage-Torque Constant (N.m/V)
K_yp = K_t_p / R_m_p;
K_py = K_t_y / R_m_y;

% Pitch and Yaw Viscous Damping Constant (N.m.s/rad)
B_p = 0.8;  % tuned while running simulation and experiment in parallel
B_y = 0.318; % identified as described in manual 

% Mass of the Helicopter (kg)
m_heli = 1.3872;

% Mass of the Helicopter with Yoke (kg)
m_heli_case = 1.421;

% Distance from Pitch Pivot to Pitch/Front Motor and Yaw/Back Motor(m)
r_p = 7.75*0.0254;
r_y = (6+5/8)*0.0254;

% Pitch and Yaw Propeller Force-Thrust Constant found Experimentally (N/V)
K_f_p = 5*0.2074;
K_f_y = 3*0.1426;

% Pitch and Yaw Propeller Torque-Thrust Constant found Experimentally (N.m/V)
K_pp = K_f_p * r_p;
K_yy = K_f_y * r_y;

% Mass of Pitch/Front Motor and Yaw/Back Motor (kg)
m_motor_p = 0.292;
m_motor_y = 0.128;

% Mass of Pitch/Front and Yaw/Back Guard + Propeller(kg)
m_shield = 0.143 + 0.024;

% Total Mass of Pitch and Yaw Motor/Shield Assemblies (kg)
m_props = ( m_motor_p + m_motor_y + 2 * m_shield );

% Mass of Helicopter Body moving about Pitch Axis (kg)
m_body_p = m_heli - m_props; 

% Mass of Helicopter Body moving about Yaw Axis (kg)
m_body_y = m_heli_case - m_props; 

% Mass of Metal Shaft Moving about Yaw Axis (kg)
m_shaft = 0.151;

% Total Length of Helicopter Body (m)
L_body = 19*0.0254;

% Helicopter Center of Mass from Pivot along Pitch Axis (m)
l_cm = ( (m_motor_p + m_shield ) * r_p +  (m_motor_y + m_shield ) * r_y ) / ( m_props ) ;

% Length of Metal Shaft Moving about Yaw Axis through slip ring (m)
L_shaft = 11 * 0.0254;

% Pitch and Yaw Motor Rotor Moment of Inertia (kg.m^2)
J_m_p = 1.91e-6; %1.7070e-5;
J_m_y = 1.374e-4; %1.4471e-5;

% Moment of Inertia of Helicopter Body about its CM (kg.m^2)
J_body_p = m_body_p * L_body^2 / 12;
J_body_y = m_body_y * L_body^2 / 12;

% Moment of Inertia of Metal Shaft about Yaw Axis (kg.m^2)
J_shaft = m_shaft * L_shaft^2 / 3; %;0.0851;

% Moment of Inertia of Pitch Motor + Guard Assembly about Pivot (kg.m^2)
J_p = ( m_motor_p + m_shield ) * r_p^2;

% Moment of Inertia of Yaw Motor + Guard Assembly about Pivot (kg.m^2)
J_y = ( m_motor_y + m_shield ) * r_y^2;

% Equivalent Moment of Inertia about Pitch and Yaw Axis (kg.m^2)
J_eq_p = J_m_p + J_body_p + J_p + J_y;
J_eq_y = J_m_y + J_body_y + J_p + J_y + J_shaft;
%%
%%
xd=0
 dx1=x3;
dx2=x4;
dx3=(1/(J_eq_p +m_heli*l_cm^2))*((K_pp*u1+K_py*u2)-(B_p*x3+m_heli*l_cm^2*x4^2*sin(x1)*cos(x1)+m_heli*g*l_cm*cos(x1)));
dx3=dx3+xd;
dx4=1/(J_eq_y + m_heli *l_cm^2* (cos(x1))^2 )*((K_yp*u1 )+(K_yy*u2 ))+(-B_y*x4+2*m_heli*l_cm^2*x4*x3*sin(x1)*cos(x1))/(J_eq_p+ m_heli * l_cm^2 * (cos(x1))^2);

== matlab function Integral_controller_disturbance/Disturbance ==
  data: xw1 input; dxw1 output; xw2 input; dxw2 output; w output; uw input
function [dxw1,dxw2,w] = Disturbance(xw1,xw2,uw)

Aw = [0 1;-4 -4];
xw = [xw1;xw2]+[0;1]*uw;
dxw = Aw*xw;
dxw1 = dxw(1);
dxw2 = dxw(2);
Cw = [1 0;0 1];
w = Cw*xw;
